simulink model "zxy3_1"  (R2017b)
settings: Solver=VariableStepAuto  StartTime=0.0  StopTime=100  RelTol=1e-3
settings Model: Creator=zxy19  LastModifiedBy=zxy19

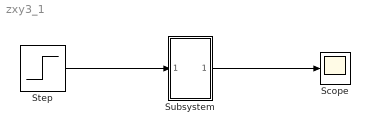
== system zxy3_1 ==
  Scope : Scope
  Step : Step  SampleTime=0
  Subsystem : Subsystem  mask{Kp=0.54, Ti=8, Td=0.228}
  wires:
  Step/1 -> Subsystem/1(In1)
  Subsystem/1(Out1) -> Scope/1

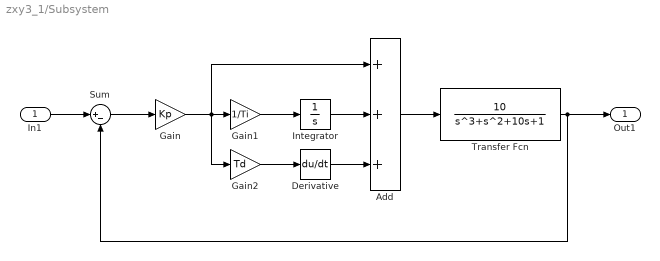
== system zxy3_1/Subsystem ==
  In1 : Inport
  Add : Sum  Inputs=+++
  Derivative : Derivative
  Gain : Gain  Gain=Kp
  Gain1 : Gain  Gain=1/Ti
  Gain2 : Gain  Gain=Td
  Integrator : Integrator
  Sum : Sum  Inputs=|+-
  Transfer Fcn : TransferFcn  Numerator=[10]  Denominator=[1 1 10 1]
  Out1 : Outport
  wires:
  Derivative/1 -> Add/3
  Integrator/1 -> Add/2
  Add/1 -> Transfer Fcn/1
  Gain/1 -> Add/1, Gain2/1, Gain1/1
  Gain1/1 -> Integrator/1
  Gain2/1 -> Derivative/1
  In1/1 -> Sum/1
  Sum/1 -> Gain/1
  Transfer Fcn/1 -> Out1/1, Sum/2
